simulink model "rslqr"  (R2021a)
settings: Solver=FixedStepAuto  StartTime=0.0  StopTime=10  RelTol=1e-3
values from neighbouring files (symbols this model uses):
  F = 100    [setup_env.m]    (also in setup_env_5_4.m)
undefined symbols (not defined in the file or in its folder): sslist, trimlist
libraries: dspsigops x2, cstblocks x1
settings Model: Creator=seedship  LastModifiedBy=seedship
settings SolverCC: AlgebraicLoopSolver=TrustRegion
settings OptimizationCC: ZeroExternalMemoryAtStartup=off  ZeroInternalMemoryAtStartup=off  InitFltsAndDblsToZero=on
settings DebuggingCC: SFMachineParentedDataDiag=warning
settings HardwareCC: ProdBitPerLong=64  ProdLongLongMode=on  ProdHWDeviceType=Intel->x86-64 (Linux 64)  TargetLongLongMode=on
settings RTWCC: BuildConfiguration=Faster Runs  TargetLang=C++  GenerateGPUCode=CUDA
settings GRTTargetCC: TargetLangStandard=C++03 (ISO)  CodeInterfacePackaging=C++ class

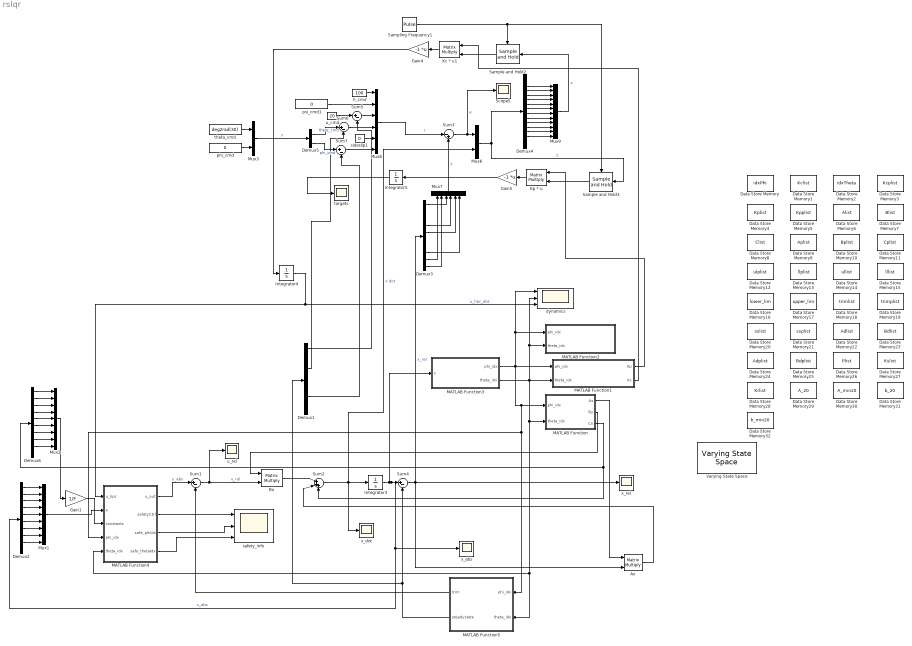
== system rslqr ==
  Ax : Product  Multiplication=Matrix(*)
  Bu : Product  Multiplication=Matrix(*)
  Data Store Memory : DataStoreMemory  DataStoreName=idxPhi  ReadBeforeWriteMsg=warning  WriteAfterWriteMsg=warning  WriteAfterReadMsg=warning  InitialValue=idxPhi  VectorParams1D=off  ShowAdditionalParam=off  OutDataTypeStr=double
  Data Store Memory1 : DataStoreMemory  DataStoreName=Kclist  ReadBeforeWriteMsg=warning  WriteAfterWriteMsg=warning  WriteAfterReadMsg=warning  InitialValue=Kclist  VectorParams1D=off  ShowAdditionalParam=off  OutDataTypeStr=double
  Data Store Memory10 : DataStoreMemory  DataStoreName=Bplist  ReadBeforeWriteMsg=warning  WriteAfterWriteMsg=warning  WriteAfterReadMsg=warning  InitialValue=Bplist  VectorParams1D=off  ShowAdditionalParam=off  OutDataTypeStr=double
  Data Store Memory11 : DataStoreMemory  DataStoreName=Cplist  ReadBeforeWriteMsg=warning  WriteAfterWriteMsg=warning  WriteAfterReadMsg=warning  InitialValue=Cplist  VectorParams1D=off  ShowAdditionalParam=off  OutDataTypeStr=double
  Data Store Memory12 : DataStoreMemory  DataStoreName=ulplist  ReadBeforeWriteMsg=warning  WriteAfterWriteMsg=warning  WriteAfterReadMsg=warning  InitialValue=ulplist  VectorParams1D=off  ShowAdditionalParam=off  OutDataTypeStr=double
  Data Store Memory13 : DataStoreMemory  DataStoreName=llplist  ReadBeforeWriteMsg=warning  WriteAfterWriteMsg=warning  WriteAfterReadMsg=warning  InitialValue=llplist  VectorParams1D=off  ShowAdditionalParam=off  OutDataTypeStr=double
  Data Store Memory14 : DataStoreMemory  DataStoreName=ullist  ReadBeforeWriteMsg=warning  WriteAfterWriteMsg=warning  WriteAfterReadMsg=warning  InitialValue=ullist  VectorParams1D=off  ShowAdditionalParam=off  OutDataTypeStr=double
  Data Store Memory15 : DataStoreMemory  DataStoreName=lllist  ReadBeforeWriteMsg=warning  WriteAfterWriteMsg=warning  WriteAfterReadMsg=warning  InitialValue=lllist  VectorParams1D=off  ShowAdditionalParam=off  OutDataTypeStr=double
  Data Store Memory16 : DataStoreMemory  DataStoreName=lower_lim  ReadBeforeWriteMsg=warning  WriteAfterWriteMsg=warning  WriteAfterReadMsg=warning  InitialValue=lower_lim  VectorParams1D=off  ShowAdditionalParam=off  OutDataTypeStr=double
  Data Store Memory17 : DataStoreMemory  DataStoreName=upper_lim  ReadBeforeWriteMsg=warning  WriteAfterWriteMsg=warning  WriteAfterReadMsg=warning  InitialValue=upper_lim  VectorParams1D=off  ShowAdditionalParam=off  OutDataTypeStr=double
  Data Store Memory18 : DataStoreMemory  DataStoreName=trimlist  ReadBeforeWriteMsg=warning  WriteAfterWriteMsg=warning  WriteAfterReadMsg=warning  InitialValue=trimlist  VectorParams1D=off  ShowAdditionalParam=off  OutDataTypeStr=double
  Data Store Memory19 : DataStoreMemory  DataStoreName=trimplist  ReadBeforeWriteMsg=warning  WriteAfterWriteMsg=warning  WriteAfterReadMsg=warning  InitialValue=trimplist  VectorParams1D=off  ShowAdditionalParam=off  OutDataTypeStr=double
  Data Store Memory2 : DataStoreMemory  DataStoreName=idxTheta  ReadBeforeWriteMsg=warning  WriteAfterWriteMsg=warning  WriteAfterReadMsg=warning  InitialValue=idxTheta  ShowAdditionalParam=off  OutDataTypeStr=double
  Data Store Memory20 : DataStoreMemory  DataStoreName=sslist  ReadBeforeWriteMsg=warning  WriteAfterWriteMsg=warning  WriteAfterReadMsg=warning  InitialValue=sslist  VectorParams1D=off  ShowAdditionalParam=off  OutDataTypeStr=double
  Data Store Memory21 : DataStoreMemory  DataStoreName=ssplist  ReadBeforeWriteMsg=warning  WriteAfterWriteMsg=warning  WriteAfterReadMsg=warning  InitialValue=ssplist  VectorParams1D=off  ShowAdditionalParam=off  OutDataTypeStr=double
  Data Store Memory22 : DataStoreMemory  DataStoreName=Adlist  ReadBeforeWriteMsg=warning  WriteAfterWriteMsg=warning  WriteAfterReadMsg=warning  InitialValue=Adlist  VectorParams1D=off  ShowAdditionalParam=off  OutDataTypeStr=double
  Data Store Memory23 : DataStoreMemory  DataStoreName=Bdlist  ReadBeforeWriteMsg=warning  WriteAfterWriteMsg=warning  WriteAfterReadMsg=warning  InitialValue=Bdlist  VectorParams1D=off  ShowAdditionalParam=off  OutDataTypeStr=double
  Data Store Memory24 : DataStoreMemory  DataStoreName=Adplist  ReadBeforeWriteMsg=warning  WriteAfterWriteMsg=warning  WriteAfterReadMsg=warning  InitialValue=Adplist  VectorParams1D=off  ShowAdditionalParam=off  OutDataTypeStr=double
  Data Store Memory25 : DataStoreMemory  DataStoreName=Bdplist  ReadBeforeWriteMsg=warning  WriteAfterWriteMsg=warning  WriteAfterReadMsg=warning  InitialValue=Bdplist  VectorParams1D=off  ShowAdditionalParam=off  OutDataTypeStr=double
  Data Store Memory26 : DataStoreMemory  DataStoreName=Plist  ReadBeforeWriteMsg=warning  WriteAfterWriteMsg=warning  WriteAfterReadMsg=warning  InitialValue=Plist  VectorParams1D=off  ShowAdditionalParam=off  OutDataTypeStr=double
  Data Store Memory27 : DataStoreMemory  DataStoreName=Kslist  ReadBeforeWriteMsg=warning  WriteAfterWriteMsg=warning  WriteAfterReadMsg=warning  InitialValue=Kslist  VectorParams1D=off  ShowAdditionalParam=off  OutDataTypeStr=double
  Data Store Memory28 : DataStoreMemory  DataStoreName=Krlist  ReadBeforeWriteMsg=warning  WriteAfterWriteMsg=warning  WriteAfterReadMsg=warning  InitialValue=Krlist  VectorParams1D=off  ShowAdditionalParam=off  OutDataTypeStr=double
  Data Store Memory29 : DataStoreMemory  DataStoreName=A_20  ReadBeforeWriteMsg=warning  WriteAfterWriteMsg=warning  WriteAfterReadMsg=warning  InitialValue=A_20  VectorParams1D=off  ShowAdditionalParam=off  OutDataTypeStr=double
  Data Store Memory3 : DataStoreMemory  DataStoreName=Kcplist  ReadBeforeWriteMsg=warning  WriteAfterWriteMsg=warning  WriteAfterReadMsg=warning  InitialValue=Kcplist  ShowAdditionalParam=off  OutDataTypeStr=double
  Data Store Memory30 : DataStoreMemory  DataStoreName=A_min20  ReadBeforeWriteMsg=warning  WriteAfterWriteMsg=warning  WriteAfterReadMsg=warning  InitialValue=A_min20  VectorParams1D=off  ShowAdditionalParam=off  OutDataTypeStr=double
  Data Store Memory31 : DataStoreMemory  DataStoreName=b_20  ReadBeforeWriteMsg=warning  WriteAfterWriteMsg=warning  WriteAfterReadMsg=warning  InitialValue=b_20  VectorParams1D=off  ShowAdditionalParam=off  OutDataTypeStr=double
  Data Store Memory32 : DataStoreMemory  DataStoreName=b_min20  ReadBeforeWriteMsg=warning  WriteAfterWriteMsg=warning  WriteAfterReadMsg=warning  InitialValue=b_min20  VectorParams1D=off  ShowAdditionalParam=off  OutDataTypeStr=double
  Data Store Memory4 : DataStoreMemory  DataStoreName=Kplist  ReadBeforeWriteMsg=warning  WriteAfterWriteMsg=warning  WriteAfterReadMsg=warning  InitialValue=Kplist  ShowAdditionalParam=off  OutDataTypeStr=double
  Data Store Memory5 : DataStoreMemory  DataStoreName=Kpplist  ReadBeforeWriteMsg=warning  WriteAfterWriteMsg=warning  WriteAfterReadMsg=warning  InitialValue=Kpplist  ShowAdditionalParam=off  OutDataTypeStr=double
  Data Store Memory6 : DataStoreMemory  DataStoreName=Alist  ReadBeforeWriteMsg=warning  WriteAfterWriteMsg=warning  WriteAfterReadMsg=warning  InitialValue=Alist  VectorParams1D=off  ShowAdditionalParam=off  OutDataTypeStr=double
  Data Store Memory7 : DataStoreMemory  DataStoreName=Blist  ReadBeforeWriteMsg=warning  WriteAfterWriteMsg=warning  WriteAfterReadMsg=warning  InitialValue=Blist  VectorParams1D=off  ShowAdditionalParam=off  OutDataTypeStr=double
  Data Store Memory8 : DataStoreMemory  DataStoreName=Clist  ReadBeforeWriteMsg=warning  WriteAfterWriteMsg=warning  WriteAfterReadMsg=warning  InitialValue=Clist  VectorParams1D=off  ShowAdditionalParam=off  OutDataTypeStr=double
  Data Store Memory9 : DataStoreMemory  DataStoreName=Aplist  ReadBeforeWriteMsg=warning  WriteAfterWriteMsg=warning  WriteAfterReadMsg=warning  InitialValue=Aplist  VectorParams1D=off  ShowAdditionalParam=off  OutDataTypeStr=double
  Demux{1..3,6} (4 alike) : Demux  Outputs=10
  Demux4 : Demux  Outputs=16
  Demux5 : Demux  Outputs=2
  Gain1 : Gain  Gain=1/F
  Gain4 : Gain  Gain=-1  Multiplication=Matrix(K*u)
  Gain5 : Gain  Gain=-1  Multiplication=Matrix(K*u)
  Integrator3 : Integrator  InitialCondition=sslist(:,3)
  Integrator4 : Integrator  InitialCondition=trimlist(:,3)  LimitOutput=on  UpperSaturationLimit=[1 1 1 1]  LowerSaturationLimit=[ -1 -1 -1 -1]
  Integrator5 : Integrator  LimitOutput=on  UpperSaturationLimit=[deg2rad(50); deg2rad(70)]  LowerSaturationLimit=[-deg2rad(50); -deg2rad(70)]
  Kc * u1 : Product  Multiplication=Matrix(*)
  Kp * u : Product  Multiplication=Matrix(*)
  MATLAB Function : MATLAB Function  TreatAsAtomicUnit=on
  MATLAB Function1 : MATLAB Function  TreatAsAtomicUnit=on
  MATLAB Function2 : MATLAB Function  TreatAsAtomicUnit=on
  MATLAB Function3 : MATLAB Function  TreatAsAtomicUnit=on
  MATLAB Function4 : MATLAB Function  TreatAsAtomicUnit=on
  MATLAB Function5 : MATLAB Function  TreatAsAtomicUnit=on
  Mux1 : Mux  Inputs=9
  Mux2 : Mux  Inputs=9
  Mux3 : Mux  Inputs=2
  Mux6 : Mux  Inputs=2
  Mux7 : Mux  Inputs=6
  Mux8 : Mux  Inputs=6
  Mux9 : Mux  Inputs=12
  Sample and Hold2 : dspsigops/Sample and Hold  trig=Rising edge  initCond=0  latchinput=off
  Sample and Hold3 : dspsigops/Sample and Hold  trig=Rising edge  initCond=0  latchinput=off
  Sampling Frequency1 : DiscretePulseGenerator  PulseType=Time based  Period=1/F  PulseWidth=50
  Scope5 : Scope
  Sum{1,4..7} (5 alike) : Sum  Inputs=|+-
  Sum2 : Sum  Inputs=|+++
  Sum3 : Sum  Inputs=|-+
  Varying State Space : cstblocks/Linear Parameter Varying/Varying State Space  x0=0  xNames=''  OutputX=on  OutputDX=on
  dynamics : Scope  NumInputPorts=3
  h_cmd : Constant  Value=100
  phi_cmd : Constant  Value=0
  psi_cmd1 : Constant  Value=0
  safety_info : Scope  NumInputPorts=3
  sideslip1 : Constant  Value=0
  targets : Scope
  theta_cmd : Constant  Value=deg2rad(30)
  u_cmd : Constant  Value=20
  u_rel : Scope
  x_abs : Scope
  x_dot : Scope
  x_rel : Scope
  wires:
  Ax/1 -> Sum2/2
  MATLAB Function/2(Bs) -> Bu/1
  Bu/1 -> Sum2/1
  MATLAB Function/3(Cs) -> Demux6/1, Sum2/3
  Mux7/1 -> Sum3/2  "y"
  Demux4/4 -> Mux9/2
  Demux4/9 -> Mux9/7
  Demux3/10 -> Mux7/2
  Sum3/1 -> Scope5/1, Mux6/1  "e"
  Demux4/12 -> Mux9/10
  Demux3/9 -> Mux7/1
  h_cmd/1 -> Mux8/1
  Demux3/4 -> Mux7/4
  Demux3/1 -> Mux7/3
  Kc * u1/1 -> Gain4/1
  Demux5/2 -> Sum7/1  "phi_cmd"
  u_cmd/1 -> Sum5/1
  psi_cmd1/1 -> Mux8/2
  sideslip1/1 -> Mux8/5
  Demux4/5 -> Mux9/3
  Mux6/1 -> Sample and Hold3/1, Demux4/1  "z"
  Sampling Frequency1/1 -> Sample and Hold3/Trigger, Sample and Hold2/Trigger
  Sample and Hold2/1 -> Kc * u1/2
  Mux9/1 -> Sample and Hold2/1  "z"
  Demux3/5 -> Mux7/5
  Mux8/1 -> Sum3/1  "r"
  Demux4/13 -> Mux9/11
  Demux3/8 -> Mux7/6
  Sum2/1 -> Mux6/2, Integrator3/1, x_dot/1  "x dot"
  Demux5/1 -> Sum6/1  "theta_cmd"
  Demux4/10 -> Mux9/8
  Demux4/7 -> Mux9/5
  Demux4/8 -> Mux9/6
  Demux4/11 -> Mux9/9
  Demux4/3 -> Mux9/1
  Demux4/14 -> Mux9/12
  Demux4/6 -> Mux9/4
  Integrator5/1 -> targets/1
  Integrator4/1 -> MATLAB Function4/1(u_hpc), dynamics/3  "u_hpc_abs"
  Kp * u/1 -> Gain5/1
  Sample and Hold3/1 -> Kp * u/2
  Gain5/1 -> Integrator5/1
  Gain4/1 -> Integrator4/1
  MATLAB Function1/1(Kp) -> Kp * u/1
  MATLAB Function1/2(Kc) -> Kc * u1/1
  MATLAB Function/1(As) -> Ax/1
  MATLAB Function3/1(phi_idx) -> dynamics/1, MATLAB Function2/1(phi_idx), MATLAB Function1/1(phi_idx), MATLAB Function5/1(phi_idx), MATLAB Function4/4(phi_idx), MATLAB Function/1(phi_idx)
  MATLAB Function3/2(theta_idx) -> dynamics/2, MATLAB Function2/2(theta_idx), MATLAB Function1/2(theta_idx), MATLAB Function5/2(theta_idx), MATLAB Function4/5(theta_idx), MATLAB Function/2(theta_idx)
  Sum1/1 -> u_rel/1, Bu/2  "u_rel"
  MATLAB Function5/2(steadystate) -> Demux1/1, Sum4/2
  Integrator3/1 -> Demux2/1, x_abs/1, Sum4/1, MATLAB Function3/1(x)  "x_abs"
  Sum4/1 -> x_rel/1, Demux3/1, Ax/2  "x_rel"
  Sum5/1 -> Mux8/3
  Sum6/1 -> Mux8/4
  Sum7/1 -> Mux8/6
  Demux1/1 -> Sum5/2
  Demux1/4 -> Sum6/2
  Demux1/8 -> Sum7/2
  MATLAB Function5/1(trim) -> Sum1/2
  MATLAB Function4/2(safetyCtrl) -> safety_info/1
  Gain1/1 -> MATLAB Function4/3(constants)
  Demux2/1 -> Mux1/1
  Demux2/2 -> Mux1/2
  Demux2/3 -> Mux1/3
  Demux2/4 -> Mux1/4
  Demux2/5 -> Mux1/5
  Demux2/6 -> Mux1/6
  Demux2/7 -> Mux1/7
  Demux2/8 -> Mux1/8
  Demux2/9 -> Mux1/9
  Mux1/1 -> MATLAB Function4/2(x)
  Demux6/6 -> Mux2/6
  Demux6/2 -> Mux2/2
  Demux6/7 -> Mux2/7
  Demux6/8 -> Mux2/8
  Demux6/3 -> Mux2/3
  Demux6/4 -> Mux2/4
  Demux6/5 -> Mux2/5
  Demux6/9 -> Mux2/9
  Demux6/1 -> Mux2/1
  Mux2/1 -> Gain1/1
  MATLAB Function4/1(u_out) -> Sum1/1  "u_abs"
  MATLAB Function4/3(safe_phiIdx) -> safety_info/2
  MATLAB Function4/4(safe_thetaIdx) -> safety_info/3
  theta_cmd/1 -> Mux3/1
  phi_cmd/1 -> Mux3/2
  Mux3/1 -> Demux5/1  "y"

== matlab function rslqr/MATLAB Function5 ==
  settings: updateMethod=DISCRETE
  data: phi_idx input; trim output size=4; steadystate output size=10; theta_idx input; trimlist data_store_memory; trimplist data_store_memory; sslist data_store_memory; ssplist data_store_memory
function [trim, steadystate] = calculateTrimSteadyState(phi_idx, theta_idx)
    % Nearest A, B
    global trimlist trimplist sslist ssplist;
    
    if theta_idx ~= 2
        trim = trimplist(:, theta_idx);
        steadystate = ssplist(:, theta_idx);
        return
    end
    
    trim = trimlist(:, phi_idx);
    steadystate = sslist(:, phi_idx);
end

== matlab function rslqr/MATLAB Function1 ==
  settings: updateMethod=DISCRETE
  data: phi_idx input; Kclist data_store_memory; Kplist data_store_memory; Kcplist data_store_memory; Kpplist data_store_memory; Kp output size=[2 16]; Kc output size=[4 12]; theta_idx input
function [Kp,Kc] = calculateRSLQRGains(phi_idx, theta_idx)
    % Nearest A, B
    global Kclist Kplist Kcplist Kpplist
    
    
    if theta_idx ~= 2
        Kc = Kcplist(:,:, theta_idx);
        Kp = Kpplist(:,:, theta_idx);
        return
    end
    
    Kc = Kclist(:,:, phi_idx);
    Kp = Kplist(:,:, phi_idx);
end

== matlab function rslqr/MATLAB Function ==
  settings: updateMethod=DISCRETE
  data: phi_idx input; Alist data_store_memory; Aplist data_store_memory; Blist data_store_memory; Bplist data_store_memory; Clist data_store_memory; Cplist data_store_memory; As output size=[10 10]; Bs output size=[10 4]; Cs output size=10; theta_idx input
function [As,Bs, Cs] = calculateDynamics(phi_idx, theta_idx)
    % Nearest A, B
    global Alist Blist Clist Aplist Bplist Cplist;
    
    if theta_idx ~= 2
        As = Aplist(:,:, theta_idx);
        Bs = Bplist(:,:, theta_idx);
        Cs = Cplist(:, theta_idx);
        return
    end
    
    As = Alist(:,:, phi_idx);
    Bs = Blist(:,:, phi_idx);
    Cs = Clist(:, phi_idx);
end

== matlab function rslqr/MATLAB Function2 ==
  settings: updateMethod=DISCRETE
  data: phi_idx input; lllist data_store_memory; llplist data_store_memory; lower_lim data_store_memory; ullist data_store_memory; ulplist data_store_memory; upper_lim data_store_memory; theta_idx input
function setSaturation(phi_idx, theta_idx)
    % Nearest A, B
    global ullist lllist ulplist llplist upper_lim lower_lim
    
    if theta_idx ~= 2
        upper_lim = ulplist(:, theta_idx);
        lower_lim = llplist(:, theta_idx);
        return
    end
    
    upper_lim = ullist(:, phi_idx);
    lower_lim = lllist(:, phi_idx);
end

== matlab function rslqr/MATLAB Function3 ==
  settings: updateMethod=DISCRETE
  data: x input; idxPhi data_store_memory; idxTheta data_store_memory; phi_idx output size=1; theta_idx output size=1
function [phi_idx, theta_idx]= calculateIdx(x)
    % Nearest A, B
    global idxPhi idxTheta
    [~, phi_idx] = min(abs(x(8) - idxPhi));
    [~, theta_idx] = min(abs(x(4) - idxTheta));
end

== matlab function rslqr/MATLAB Function4 ==
  settings: updateMethod=DISCRETE
  data: u_hpc input; x input; constants input; u_out output; safetyCtrl output; phi_idx input; theta_idx input; Adlist data_store_memory; Adplist data_store_memory; Bdlist data_store_memory; Bdplist data_store_memory; sslist data_store_memory; ssplist data_store_memory; Plist data_store_memory; Krlist data_store_memory; Kslist data_store_memory; trimlist data_store_memory; trimplist data_store_memory; A_20 data_store_memory; A_min20 data_store_memory; b_20 data_store_memory; b_min20 data_store_memory; safe_phiIdx output; safe_thetaIdx output
function [u_out, safetyCtrl, safe_phiIdx, safe_thetaIdx] = decision_logic(u_hpc, x, constants, phi_idx, theta_idx)

    global Adlist Adplist Bdlist Bdplist sslist ssplist trimlist trimplist Plist Kslist Krlist A_20 A_min20 b_20 b_min20
    persistent lastPhiIdx lastThetaIdx safetyActivated

    if isempty(lastPhiIdx)
        lastPhiIdx = 3;
    end

    if isempty(lastThetaIdx)
        lastThetaIdx = -1;
    end

    if isempty(safetyActivated)
        safetyActivated = 0;
    end

    if theta_idx ~= 2
        % Handle pitch reachability
        nextState = Adplist(:,:,theta_idx) * (x - ssplist(1:9, theta_idx)) + Bdplist(:,:,theta_idx) * (u_hpc - trimplist(:, theta_idx)) + constants + ssplist(1:9, theta_idx);
    else
        nextState = Adlist(:,:,phi_idx) * (x - sslist(1:9, phi_idx)) + Bdlist(:,:,phi_idx) * (u_hpc - trimlist(:, phi_idx)) + constants + sslist(1:9, phi_idx);
    end

    [safe, safePhiIdx, safeThetaIdx] = nextStateInRecoverableRegion(nextState, sslist, ssplist, Plist, A_20, A_min20, b_20, b_min20);
    
    if safe
        lastPhiIdx = safePhiIdx;
        lastThetaIdx = safeThetaIdx;
    end

    % Calculate if safety control necessary
    if ~safe || safetyActivated
        % Apply safety controller
        safetyCtrl = 1;
        safetyActivated = 1;
        if lastPhiIdx ~= -1
            u_out = bound(-Kslist(:,:,lastPhiIdx) * (x - sslist(1:9, lastPhiIdx)), -1, 1) + trimlist(:, lastPhiIdx);
        elseif lastThetaIdx == 1 || lastThetaIdx == 3
            u_out = bound(-Krlist(:,:,lastThetaIdx) * (x - ssplist(1:9, lastThetaIdx)), -1, 1) + trimplist(:, lastThetaIdx);
        else
            error('Error! lastThetaIdx: %i\n', lastThetaIdx)
        end 
    else
        % apply HPC
        u_out = u_hpc;
        safetyCtrl = 0;
    end
    safe_phiIdx = lastPhiIdx;
    safe_thetaIdx = lastThetaIdx;
end

function [safe, safePhiIdx, safeThetaIdx] = nextStateInRecoverableRegion(s, sslist, ssplist, Plist, A_20, A_min20, b_20, b_min20)
    %% Test roll controllers
    safe = 0;
    safePhiIdx = -1;
    safeThetaIdx = -1;
    for idx = [3,2,4,1,5]
        x_hat = s - sslist(1:9, idx);
        if x_hat' * Plist(:,:,idx) * x_hat < 1
            safe = 1;
            safePhiIdx = idx;
%             if idx == 3
%                 safeThetaIdx = 2;
%             end
            return
        end
    end
    
    %% Test pitch reachability +20 deg
    x_hat = s - ssplist(1:9, 3);
    if contains(A_20, b_20, x_hat)
       safe = 1;
       safeThetaIdx = 3;
    end
    
    %% Test pitch reachability -20 deg
    x_hat = s - ssplist(1:9, 1);
    if contains(A_min20, b_min20, x_hat)
       safe = 1;
       safeThetaIdx = 1;
    end
    
end

function ret = contains(polyA, polyb, point)
    ret = 0;
    shape = size(polyA);
    for idx = 1:shape(3)
        if min(polyA(:,:,idx) * point <= polyb(:,idx))
            ret = 1;
            return
        end
    end
end

function y = bound(x,bl,bu)
  % return bounded value clipped between bl and bu
  y=min(max(x,bl),bu);
end
